simulink model "Phase_Control_K1"  (R2018b)
settings: Solver=VariableStepAuto  StartTime=0.0  StopTime=200  RelTol=1e-3
values from neighbouring files (symbols this model uses):
  alpha = 0.5736    [constants.m]
  c_damp = 0.00495    [constants.m]
  in_nu = 0.0001    [constants.m]
  J_r = 0.0004    [constants.m]
  J_s = 31.38    [constants.m]
  w_mode = 2.6268    [constants.m]
settings Model: Creator=Yavuz  LastModifiedBy=Yavuz
settings DebuggingCC: AlgebraicLoopMsg=none

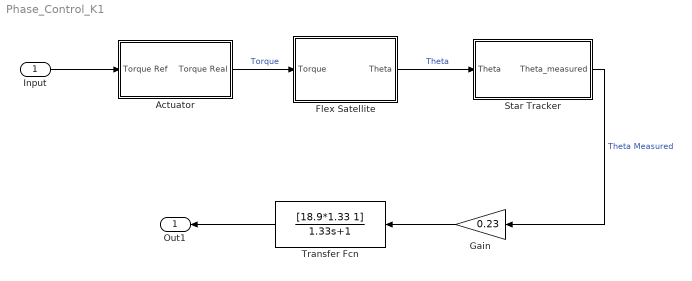
== system Phase_Control_K1 ==
  Input : Inport
  Actuator : Subsystem
  Flex Satellite : Subsystem
  Gain : Gain  Gain=0.23
  Star Tracker : Subsystem
  Transfer Fcn : TransferFcn  Numerator=[18.9*1.33 1]  Denominator=[1.33 1]
  Out1 : Outport
  wires:
  Actuator/1(Torque Real) -> Flex Satellite/1(Torque)  "Torque"
  Flex Satellite/1(Theta) -> Star Tracker/1(Theta)  "Theta"
  Input/1 -> Actuator/1(Torque Ref)
  Star Tracker/1(Theta_measured) -> Gain/1  "Theta Measured"
  Gain/1 -> Transfer Fcn/1
  Transfer Fcn/1 -> Out1/1

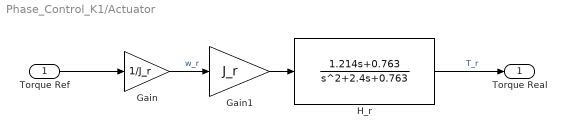
== system Phase_Control_K1/Actuator ==
  Torque Ref : Inport
  Gain : Gain  Gain=1/J_r
  Gain1 : Gain  Gain=J_r
  H_r : TransferFcn  Numerator=[1.214 0.763]  Denominator=[1 2.4 0.763]
  Torque Real : Outport
  wires:
  Torque Ref/1 -> Gain/1
  Gain1/1 -> H_r/1
  H_r/1 -> Torque Real/1  "T_r"
  Gain/1 -> Gain1/1  "w_r"

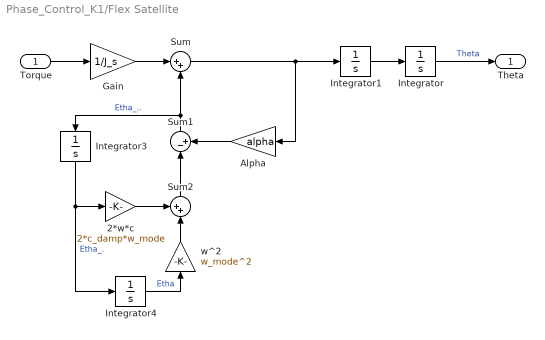
== system Phase_Control_K1/Flex Satellite ==
  Torque : Inport
  2*w*c : Gain  Gain=2*c_damp*w_mode
  Alpha : Gain  Gain=alpha
  Gain : Gain  Gain=1/J_s
  Integrator : Integrator
  Integrator1 : Integrator
  Integrator3 : Integrator
  Integrator4 : Integrator  InitialCondition=in_nu
  Sum : Sum  Inputs=|++
  Sum1 : Sum  Inputs=|-+
  Sum2 : Sum  Inputs=++|
  w^2 : Gain  Gain=w_mode^2
  Theta : Outport
  wires:
  Sum/1 -> Integrator1/1, Alpha/1
  Sum1/1 -> Integrator3/1, Sum/2  "Etha_.."
  Gain/1 -> Sum/1
  Integrator1/1 -> Integrator/1
  Integrator3/1 -> Integrator4/1, 2*w*c/1  "Etha_."
  Sum2/1 -> Sum1/1
  Torque/1 -> Gain/1
  2*w*c/1 -> Sum2/1
  Integrator/1 -> Theta/1  "Theta"
  w^2/1 -> Sum2/2
  Integrator4/1 -> w^2/1  "Etha"
  Alpha/1 -> Sum1/2

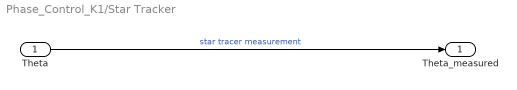
== system Phase_Control_K1/Star Tracker ==
  Theta : Inport
  Theta_measured : Outport
  wires:
  Theta/1 -> Theta_measured/1  "star tracer measurement"
